simulink model "sysgenMRIDemo"  (Simulink 7.7)
settings: Solver=VariableStepDiscrete  StartTime=0.0  StopTime=inf  RelTol=1e-3
PreLoadFcn:
  | sysgenMRIDemo_PreloadFcn
InitFcn:
  | xlFrameDisplay;
undefined symbols (not defined in the file or in its folder): a, b, c_image_cols, c_image_rows, c_num_fstores, c_swathe_size, sysgenMRIDemo_data_imag_channel, xlFrameDisplay
libraries: xbsIndex_r4 x297, dspsrcs4 x3, xbsCopyrightNotice_r4 x1, simulink x1
(part 3 of 3)

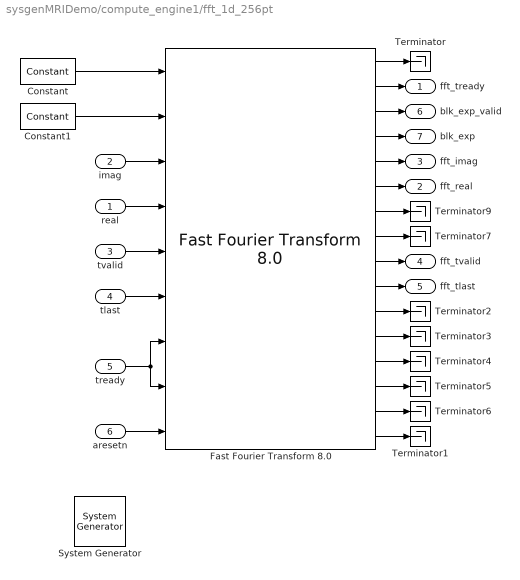
== system sysgenMRIDemo/compute_engine1/fft_1d_256pt ==
  real : Inport
  imag : Inport  Port=2
  tvalid : Inport  Port=3
  tlast : Inport  Port=4
  tready : Inport  Port=5
  aresetn : Inport  Port=6
  " System Generator" : xbsIndex_r4/ System Generator  Tag=genX  SystemSampleTime=-1  xilinxfamily=virtex6  part=xc6vlx240t  speed=-1  package=ff1156  synthesis_tool=XST  clock_wrapper=Clock Enables  directory=./netlist  proj_type=Project Navigator  Synth_file=XST Defaults  Impl_file=ISE Defaults  testbench=off  simulink_period=1  sysclk_period=10  dcm_input_clock_period=10  incr_netlist=off  trim_vbits=Everywhere in SubSystem  dbl_ovrd=According to Block Masks  core_generation=According to Block Masks  run_coregen=off  deprecated_control=off  eval_field=0  block_type=sysgen
      settings: block_version=12.3
  Constant : xbsIndex_r4/Constant  const=1  gui_display_data_type=Fixed-point  arith_type=Unsigned  n_bits=1  bin_pt=0  preci_type=Single  exp_width=8  frac_width=24  explicit_period=on  period=1  equ=P=C  opselect=C  inp2=PCIN>>17  opr=+  inp1=P  carry=CIN  dbl_ovrd=off  block_type=constant
      settings: block_version=12.3
  Constant1 : xbsIndex_r4/Constant  const=0  gui_display_data_type=Fixed-point  arith_type=Boolean  n_bits=16  bin_pt=14  preci_type=Single  exp_width=8  frac_width=24  explicit_period=on  period=1  equ=P=C  opselect=C  inp2=PCIN>>17  opr=+  inp1=P  carry=CIN  dbl_ovrd=off  block_type=constant
      settings: block_version=12.3
  "Fast Fourier Transform 8.0 " : xbsIndex_r4/Fast Fourier Transform 8.0   transform_length=256  target_clock_frequency=250  target_data_throughput=250  implementation_options=automatically_select  run_time_configurable_transform_length=off  phase_factor_width=16  scaling_options=block_floating_point  rounding_modes=truncation  aclken=off  aresetn=on  cyclic_prefix_insertion=off  output_ordering=natural_order  throttle_scheme=nonrealtime  xk_index=on  ovflo=off  trim_axipin_name=on  memory_options_data=block_ram  memory_options_phase_factors=block_ram  number_of_stages_using_block_ram_for_data_and_phase_factors=3  memory_options_reorder=block_ram  memory_options_hybrid=off  complex_mult_type=use_mults_resources  butterfly_type=use_luts  channels=1  input_ordering=natural_order  input_width=16  simulation_model=fftv8_CModel:fftv8_cmodel  ip_name=Fast Fourier Transform  ip_version=8.0  dsptool_ready=true  ipcore_usecache=true  ipcore_useipmodelcache=true  wrapper_available=true  port_translation_map={ 'aclken' => 'en', 'aresetn' => 'rst'}  block_type=xfft_v8_0
      settings: block_version=12.3
  Terminator{,1..7,9} (9 alike) : Terminator
  fft_tready : Outport
  fft_real : Outport  Port=2
  fft_imag : Outport  Port=3
  fft_tvalid : Outport  Port=4
  fft_tlast : Outport  Port=5
  blk_exp_valid : Outport  Port=6
  blk_exp : Outport  Port=7
  wires:
  "Fast Fourier Transform 8.0 "/16 -> Terminator1/1
  "Fast Fourier Transform 8.0 "/15 -> Terminator6/1
  "Fast Fourier Transform 8.0 "/14 -> Terminator5/1
  "Fast Fourier Transform 8.0 "/13 -> Terminator4/1
  "Fast Fourier Transform 8.0 "/12 -> Terminator3/1
  "Fast Fourier Transform 8.0 "/11 -> Terminator2/1
  "Fast Fourier Transform 8.0 "/10 -> fft_tlast/1
  "Fast Fourier Transform 8.0 "/9 -> fft_tvalid/1
  "Fast Fourier Transform 8.0 "/8 -> Terminator7/1
  "Fast Fourier Transform 8.0 "/7 -> Terminator9/1
  "Fast Fourier Transform 8.0 "/6 -> fft_real/1
  "Fast Fourier Transform 8.0 "/5 -> fft_imag/1
  "Fast Fourier Transform 8.0 "/4 -> blk_exp/1
  "Fast Fourier Transform 8.0 "/3 -> blk_exp_valid/1
  "Fast Fourier Transform 8.0 "/2 -> fft_tready/1
  "Fast Fourier Transform 8.0 "/1 -> Terminator/1
  aresetn/1 -> "Fast Fourier Transform 8.0 "/9
  tready/1 -> "Fast Fourier Transform 8.0 "/8, "Fast Fourier Transform 8.0 "/7
  tlast/1 -> "Fast Fourier Transform 8.0 "/6
  tvalid/1 -> "Fast Fourier Transform 8.0 "/5
  real/1 -> "Fast Fourier Transform 8.0 "/4
  imag/1 -> "Fast Fourier Transform 8.0 "/3
  Constant1/1 -> "Fast Fourier Transform 8.0 "/2
  Constant/1 -> "Fast Fourier Transform 8.0 "/1

== system sysgenMRIDemo/image_Src1/Subsystem ==
  Enable : EnablePort  PropagateVarSize=During execution
  Imag Channel : dspsrcs4/Signal From Workspace  SystemSampleTime=-1  X=sysgenMRIDemo_data_imag_channel  Ts=1  nsamps=1  OutputAfterFinalValue=Setting to zero  ignoreOrWarnInputAndFrameLengths=off
  Imag Channel1 : dspsrcs4/Signal From Workspace  SystemSampleTime=-1  X=ones(1,length(sysgenMRIDemo_data_imag_channel))  Ts=1  nsamps=1  OutputAfterFinalValue=Setting to zero  ignoreOrWarnInputAndFrameLengths=off
  Real Channel : dspsrcs4/Signal From Workspace  SystemSampleTime=-1  X=sysgenMRIDemo_data_real_channel  Ts=1  nsamps=1  OutputAfterFinalValue=Setting to zero  ignoreOrWarnInputAndFrameLengths=off
  MriReal : Outport
  MriImag : Outport  Port=2
  MriDataValid : Outport  Port=3
  wires:
  Imag Channel/1 -> MriImag/1
  Real Channel/1 -> MriReal/1
  Imag Channel1/1 -> MriDataValid/1

== system sysgenMRIDemo/Provide Register Data1/MM2S and S2MM Control Register Update/VDMA_Control_Register_Addresses ==
  rst : Inport
  en : Inport  Port=2
  ROM : xbsIndex_r4/ROM  depth=length(c_sequence)  initVector=c_sequence  distributed_mem=Distributed memory  rst=off  init_reg=0  en=off  latency=0  gui_display_data_type=Fixed-point  arith_type=Unsigned  n_bits=32  bin_pt=0  preci_type=Single  exp_width=8  frac_width=24  dbl_ovrd=off  optimize=Area  use_rpm=on  block_type=sprom
      settings: block_version=12.3
  count_down1 : Subsystem  mask{init_val=length(c_sequence)-1}
      mask prompts: init_val "Initial Value"
  seq : Outport
  wires:
  count_down1/1(cnt) -> ROM/1
  rst/1 -> count_down1/1(rst)
  ROM/1 -> seq/1
  en/1 -> count_down1/2(en)

== system sysgenMRIDemo/Provide Register Data1/MM2S and S2MM Control Register Update/VDMA_Control_Register_Addresses1 ==
  rst : Inport
  en : Inport  Port=2
  ROM : xbsIndex_r4/ROM  depth=length(c_sequence)  initVector=c_sequence  distributed_mem=Distributed memory  rst=off  init_reg=0  en=off  latency=0  gui_display_data_type=Fixed-point  arith_type=Unsigned  n_bits=32  bin_pt=0  preci_type=Single  exp_width=8  frac_width=24  dbl_ovrd=off  optimize=Area  use_rpm=on  block_type=sprom
      settings: block_version=12.3
  count_down1 : Subsystem  mask{init_val=length(c_sequence)-1}
      mask prompts: init_val "Initial Value"
  seq : Outport
  wires:
  count_down1/1(cnt) -> ROM/1
  rst/1 -> count_down1/1(rst)
  ROM/1 -> seq/1
  en/1 -> count_down1/2(en)

== system sysgenMRIDemo/Provide Register Data1/MM2S and S2MM Control Register Update/pulse_gen_we ==
  d : Inport
  rst : Inport  Port=2
  en : Inport  Port=3
  Register{,1..7} (8 alike) : xbsIndex_r4/Register  init=1  rst=on  en=on  dbl_ovrd=off  block_type=register
      settings: block_version=12.3
  q : Outport
  wires:
  Register6/1 -> Register7/1
  Register5/1 -> Register6/1
  Register4/1 -> Register5/1
  Register3/1 -> Register4/1
  Register7/1 -> q/1
  Register2/1 -> Register3/1
  en/1 -> Register7/3, Register6/3, Register5/3, Register4/3, Register3/3, Register2/3, Register1/3, Register/3
  rst/1 -> Register7/2, Register6/2, Register5/2, Register4/2, Register3/2, Register2/2, Register1/2, Register/2
  d/1 -> Register/1
  Register/1 -> Register1/1
  Register1/1 -> Register2/1

== system sysgenMRIDemo/Provide Register Data1/MM2S and S2MM Control Register Update/pulse_gen_we1 ==
  d : Inport
  rst : Inport  Port=2
  en : Inport  Port=3
  Register{,1..7} (8 alike) : xbsIndex_r4/Register  init=0  rst=on  en=on  dbl_ovrd=off  block_type=register
      settings: block_version=12.3
  q : Outport
  wires:
  Register6/1 -> Register7/1
  Register5/1 -> Register6/1
  Register3/1 -> Register4/1
  Register4/1 -> Register5/1
  Register1/1 -> Register2/1
  Register/1 -> Register1/1
  d/1 -> Register/1
  rst/1 -> Register/2, Register1/2, Register7/2, Register6/2, Register5/2, Register4/2, Register3/2, Register2/2
  en/1 -> Register/3, Register1/3, Register2/3, Register3/3, Register4/3, Register5/3, Register6/3, Register7/3
  Register2/1 -> Register3/1
  Register7/1 -> q/1

== system sysgenMRIDemo/Provide Register Data1/MM2S and S2MM Control Register Update/pulse_gen_we2 ==
  d : Inport
  rst : Inport  Port=2
  en : Inport  Port=3
  Register{,1..3} (4 alike) : xbsIndex_r4/Register  init=1  rst=on  en=on  dbl_ovrd=off  block_type=register
      settings: block_version=12.3
  q : Outport
  wires:
  Register3/1 -> q/1
  Register2/1 -> Register3/1
  en/1 -> Register2/3, Register3/3, Register1/3, Register/3
  rst/1 -> Register2/2, Register3/2, Register1/2, Register/2
  d/1 -> Register/1
  Register/1 -> Register1/1
  Register1/1 -> Register2/1

== system sysgenMRIDemo/Provide Register Data1/MM2S and S2MM Control Register Update/pulse_gen_we3 ==
  d : Inport
  rst : Inport  Port=2
  en : Inport  Port=3
  Register{,1..3} (4 alike) : xbsIndex_r4/Register  init=0  rst=on  en=on  dbl_ovrd=off  block_type=register
      settings: block_version=12.3
  q : Outport
  wires:
  Register1/1 -> Register2/1
  Register/1 -> Register1/1
  d/1 -> Register/1
  rst/1 -> Register/2, Register1/2, Register2/2, Register3/2
  en/1 -> Register/3, Register1/3, Register2/3, Register3/3
  Register2/1 -> Register3/1
  Register3/1 -> q/1

== system sysgenMRIDemo/Provide Register Data1/MM2S and S2MM Control Register Update/register_sequence ==
  rst : Inport
  en : Inport  Port=2
  ROM : xbsIndex_r4/ROM  depth=length(c_sequence)  initVector=c_sequence  distributed_mem=Distributed memory  rst=off  init_reg=0  en=off  latency=0  gui_display_data_type=Fixed-point  arith_type=Unsigned  n_bits=32  bin_pt=0  preci_type=Single  exp_width=8  frac_width=24  dbl_ovrd=off  optimize=Area  use_rpm=on  block_type=sprom
      settings: block_version=12.3
  count_down1 : Subsystem  mask{init_val=length(c_sequence)-1}
      mask prompts: init_val "Initial Value"
  seq : Outport
  wires:
  count_down1/1(cnt) -> ROM/1
  rst/1 -> count_down1/1(rst)
  ROM/1 -> seq/1
  en/1 -> count_down1/2(en)

== system sysgenMRIDemo/Provide Register Data1/MM2S and S2MM Control Register Update/register_sequence1 ==
  rst : Inport
  en : Inport  Port=2
  ROM : xbsIndex_r4/ROM  depth=length(c_sequence)  initVector=c_sequence  distributed_mem=Distributed memory  rst=off  init_reg=0  en=off  latency=0  gui_display_data_type=Fixed-point  arith_type=Unsigned  n_bits=32  bin_pt=0  preci_type=Single  exp_width=8  frac_width=24  dbl_ovrd=off  optimize=Area  use_rpm=on  block_type=sprom
      settings: block_version=12.3
  count_down1 : Subsystem  mask{init_val=length(c_sequence)-1}
      mask prompts: init_val "Initial Value"
  seq : Outport
  wires:
  count_down1/1(cnt) -> ROM/1
  rst/1 -> count_down1/1(rst)
  ROM/1 -> seq/1
  en/1 -> count_down1/2(en)

== system sysgenMRIDemo/Provide Register Data1/S2MM Control Register Update/VDMA_Control_Register_Addresses ==
  rst : Inport
  en : Inport  Port=2
  ROM : xbsIndex_r4/ROM  depth=length(c_sequence)  initVector=c_sequence  distributed_mem=Distributed memory  rst=off  init_reg=0  en=off  latency=0  gui_display_data_type=Fixed-point  arith_type=Unsigned  n_bits=32  bin_pt=0  preci_type=Single  exp_width=8  frac_width=24  dbl_ovrd=off  optimize=Area  use_rpm=on  block_type=sprom
      settings: block_version=12.3
  count_down1 : Subsystem  mask{init_val=length(c_sequence)-1}
      mask prompts: init_val "Initial Value"
  seq : Outport
  wires:
  count_down1/1(cnt) -> ROM/1
  rst/1 -> count_down1/1(rst)
  ROM/1 -> seq/1
  en/1 -> count_down1/2(en)

== system sysgenMRIDemo/Provide Register Data1/S2MM Control Register Update/VDMA_Control_Register_Data2 ==
  rst : Inport
  en : Inport  Port=2
  ROM : xbsIndex_r4/ROM  depth=length(c_sequence)  initVector=c_sequence  distributed_mem=Distributed memory  rst=off  init_reg=0  en=off  latency=0  gui_display_data_type=Fixed-point  arith_type=Unsigned  n_bits=32  bin_pt=0  preci_type=Single  exp_width=8  frac_width=24  dbl_ovrd=off  optimize=Area  use_rpm=on  block_type=sprom
      settings: block_version=12.3
  count_down1 : Subsystem  mask{init_val=length(c_sequence)-1}
      mask prompts: init_val "Initial Value"
  seq : Outport
  wires:
  count_down1/1(cnt) -> ROM/1
  rst/1 -> count_down1/1(rst)
  ROM/1 -> seq/1
  en/1 -> count_down1/2(en)

== system sysgenMRIDemo/Provide Register Data1/S2MM Control Register Update/pulse_gen_re ==
  d : Inport
  rst : Inport  Port=2
  en : Inport  Port=3
  Register{,1..3} (4 alike) : xbsIndex_r4/Register  init=0  rst=on  en=on  dbl_ovrd=off  block_type=register
      settings: block_version=12.3
  q : Outport
  wires:
  Register3/1 -> q/1
  Register2/1 -> Register3/1
  Register1/1 -> Register2/1
  Register/1 -> Register1/1
  d/1 -> Register/1
  rst/1 -> Register/2, Register3/2, Register2/2, Register1/2
  en/1 -> Register/3, Register3/3, Register2/3, Register1/3

== system sysgenMRIDemo/Provide Register Data1/S2MM Control Register Update/pulse_gen_we ==
  d : Inport
  rst : Inport  Port=2
  en : Inport  Port=3
  Register{,1..3} (4 alike) : xbsIndex_r4/Register  init=1  rst=on  en=on  dbl_ovrd=off  block_type=register
      settings: block_version=12.3
  q : Outport
  wires:
  Register3/1 -> q/1
  Register2/1 -> Register3/1
  en/1 -> Register3/3, Register2/3, Register1/3, Register/3
  rst/1 -> Register3/2, Register2/2, Register1/2, Register/2
  d/1 -> Register/1
  Register/1 -> Register1/1
  Register1/1 -> Register2/1

== system sysgenMRIDemo/Provide Register Data1/MM2S and S2MM Control Register Update/VDMA_Control_Register_Addresses/count_down1 ==
  rst : Inport
  en : Inport  Port=2
  Constant3 : xbsIndex_r4/Constant  const=0  gui_display_data_type=Fixed-point  arith_type=Unsigned  n_bits=ceil(ceil( (c_image_rows/c_swathe_size) / c_num_fstores) + 1)  bin_pt=0  preci_type=Single  exp_width=8  frac_width=24  explicit_period=off  period=1  equ=P=C  opselect=C  inp2=PCIN>>17  opr=+  inp1=P  carry=CIN  dbl_ovrd=off  block_type=constant
      settings: block_version=12.3
  Counter : xbsIndex_r4/Counter  cnt_type=Count Limited  cnt_to=0  operation=Down  start_count=init_val  cnt_by_val=1  arith_type=Unsigned  n_bits=ceil(log2(init_val + 1))  bin_pt=0  load_pin=off  rst=on  en=on  explicit_period=on  period=1  dbl_ovrd=off  use_behavioral_HDL=off  implementation=Fabric  block_type=counter
      settings: block_version=12.3
  Expression : xbsIndex_r4/Expression  expression=a & b  align_bp=on  en=off  latency=0  precision=Full  arith_type=Unsigned  n_bits=16  bin_pt=0  dbl_ovrd=off  block_type=expr
      settings: block_version=12.3
  Relational1 : xbsIndex_r4/Relational  mode=a!=b  en=off  latency=0  dbl_ovrd=off  block_type=relational
      settings: block_version=12.3
  cnt : Outport
  wires:
  en/1 -> Expression/2
  Relational1/1 -> Expression/1
  Constant3/1 -> Relational1/2
  Counter/1 -> cnt/1, Relational1/1
  Expression/1 -> Counter/2
  rst/1 -> Counter/1

== system sysgenMRIDemo/Provide Register Data1/MM2S and S2MM Control Register Update/VDMA_Control_Register_Addresses1/count_down1 ==
  rst : Inport
  en : Inport  Port=2
  Constant3 : xbsIndex_r4/Constant  const=0  gui_display_data_type=Fixed-point  arith_type=Unsigned  n_bits=ceil(ceil( (c_image_rows/c_swathe_size) / c_num_fstores) + 1)  bin_pt=0  preci_type=Single  exp_width=8  frac_width=24  explicit_period=off  period=1  equ=P=C  opselect=C  inp2=PCIN>>17  opr=+  inp1=P  carry=CIN  dbl_ovrd=off  block_type=constant
      settings: block_version=12.3
  Counter : xbsIndex_r4/Counter  cnt_type=Count Limited  cnt_to=0  operation=Down  start_count=init_val  cnt_by_val=1  arith_type=Unsigned  n_bits=ceil(log2(init_val + 1))  bin_pt=0  load_pin=off  rst=on  en=on  explicit_period=on  period=1  dbl_ovrd=off  use_behavioral_HDL=off  implementation=Fabric  block_type=counter
      settings: block_version=12.3
  Expression : xbsIndex_r4/Expression  expression=a & b  align_bp=on  en=off  latency=0  precision=Full  arith_type=Unsigned  n_bits=16  bin_pt=0  dbl_ovrd=off  block_type=expr
      settings: block_version=12.3
  Relational1 : xbsIndex_r4/Relational  mode=a!=b  en=off  latency=0  dbl_ovrd=off  block_type=relational
      settings: block_version=12.3
  cnt : Outport
  wires:
  en/1 -> Expression/2
  Relational1/1 -> Expression/1
  Constant3/1 -> Relational1/2
  Counter/1 -> cnt/1, Relational1/1
  Expression/1 -> Counter/2
  rst/1 -> Counter/1

== system sysgenMRIDemo/Provide Register Data1/MM2S and S2MM Control Register Update/register_sequence/count_down1 ==
  rst : Inport
  en : Inport  Port=2
  Constant3 : xbsIndex_r4/Constant  const=0  gui_display_data_type=Fixed-point  arith_type=Unsigned  n_bits=ceil(ceil( (c_image_rows/c_swathe_size) / c_num_fstores) + 1)  bin_pt=0  preci_type=Single  exp_width=8  frac_width=24  explicit_period=off  period=1  equ=P=C  opselect=C  inp2=PCIN>>17  opr=+  inp1=P  carry=CIN  dbl_ovrd=off  block_type=constant
      settings: block_version=12.3
  Counter : xbsIndex_r4/Counter  cnt_type=Count Limited  cnt_to=0  operation=Down  start_count=init_val  cnt_by_val=1  arith_type=Unsigned  n_bits=ceil(log2(init_val + 1))  bin_pt=0  load_pin=off  rst=on  en=on  explicit_period=on  period=1  dbl_ovrd=off  use_behavioral_HDL=off  implementation=Fabric  block_type=counter
      settings: block_version=12.3
  Expression : xbsIndex_r4/Expression  expression=a & b  align_bp=on  en=off  latency=0  precision=Full  arith_type=Unsigned  n_bits=16  bin_pt=0  dbl_ovrd=off  block_type=expr
      settings: block_version=12.3
  Relational1 : xbsIndex_r4/Relational  mode=a!=b  en=off  latency=0  dbl_ovrd=off  block_type=relational
      settings: block_version=12.3
  cnt : Outport
  wires:
  en/1 -> Expression/2
  Relational1/1 -> Expression/1
  Constant3/1 -> Relational1/2
  Counter/1 -> cnt/1, Relational1/1
  Expression/1 -> Counter/2
  rst/1 -> Counter/1

== system sysgenMRIDemo/Provide Register Data1/MM2S and S2MM Control Register Update/register_sequence1/count_down1 ==
  rst : Inport
  en : Inport  Port=2
  Constant3 : xbsIndex_r4/Constant  const=0  gui_display_data_type=Fixed-point  arith_type=Unsigned  n_bits=ceil(ceil( (c_image_rows/c_swathe_size) / c_num_fstores) + 1)  bin_pt=0  preci_type=Single  exp_width=8  frac_width=24  explicit_period=off  period=1  equ=P=C  opselect=C  inp2=PCIN>>17  opr=+  inp1=P  carry=CIN  dbl_ovrd=off  block_type=constant
      settings: block_version=12.3
  Counter : xbsIndex_r4/Counter  cnt_type=Count Limited  cnt_to=0  operation=Down  start_count=init_val  cnt_by_val=1  arith_type=Unsigned  n_bits=ceil(log2(init_val + 1))  bin_pt=0  load_pin=off  rst=on  en=on  explicit_period=on  period=1  dbl_ovrd=off  use_behavioral_HDL=off  implementation=Fabric  block_type=counter
      settings: block_version=12.3
  Expression : xbsIndex_r4/Expression  expression=a & b  align_bp=on  en=off  latency=0  precision=Full  arith_type=Unsigned  n_bits=16  bin_pt=0  dbl_ovrd=off  block_type=expr
      settings: block_version=12.3
  Relational1 : xbsIndex_r4/Relational  mode=a!=b  en=off  latency=0  dbl_ovrd=off  block_type=relational
      settings: block_version=12.3
  cnt : Outport
  wires:
  en/1 -> Expression/2
  Relational1/1 -> Expression/1
  Constant3/1 -> Relational1/2
  Counter/1 -> cnt/1, Relational1/1
  Expression/1 -> Counter/2
  rst/1 -> Counter/1

== system sysgenMRIDemo/Provide Register Data1/S2MM Control Register Update/VDMA_Control_Register_Addresses/count_down1 ==
  rst : Inport
  en : Inport  Port=2
  Constant3 : xbsIndex_r4/Constant  const=0  gui_display_data_type=Fixed-point  arith_type=Unsigned  n_bits=ceil(ceil( (c_image_rows/c_swathe_size) / c_num_fstores) + 1)  bin_pt=0  preci_type=Single  exp_width=8  frac_width=24  explicit_period=off  period=1  equ=P=C  opselect=C  inp2=PCIN>>17  opr=+  inp1=P  carry=CIN  dbl_ovrd=off  block_type=constant
      settings: block_version=12.3
  Counter : xbsIndex_r4/Counter  cnt_type=Count Limited  cnt_to=0  operation=Down  start_count=init_val  cnt_by_val=1  arith_type=Unsigned  n_bits=ceil(log2(init_val + 1))  bin_pt=0  load_pin=off  rst=on  en=on  explicit_period=on  period=1  dbl_ovrd=off  use_behavioral_HDL=off  implementation=Fabric  block_type=counter
      settings: block_version=12.3
  Expression : xbsIndex_r4/Expression  expression=a & b  align_bp=on  en=off  latency=0  precision=Full  arith_type=Unsigned  n_bits=16  bin_pt=0  dbl_ovrd=off  block_type=expr
      settings: block_version=12.3
  Relational1 : xbsIndex_r4/Relational  mode=a!=b  en=off  latency=0  dbl_ovrd=off  block_type=relational
      settings: block_version=12.3
  cnt : Outport
  wires:
  en/1 -> Expression/2
  Relational1/1 -> Expression/1
  Constant3/1 -> Relational1/2
  Counter/1 -> cnt/1, Relational1/1
  Expression/1 -> Counter/2
  rst/1 -> Counter/1

== system sysgenMRIDemo/Provide Register Data1/S2MM Control Register Update/VDMA_Control_Register_Data2/count_down1 ==
  rst : Inport
  en : Inport  Port=2
  Constant3 : xbsIndex_r4/Constant  const=0  gui_display_data_type=Fixed-point  arith_type=Unsigned  n_bits=ceil(ceil( (c_image_rows/c_swathe_size) / c_num_fstores) + 1)  bin_pt=0  preci_type=Single  exp_width=8  frac_width=24  explicit_period=off  period=1  equ=P=C  opselect=C  inp2=PCIN>>17  opr=+  inp1=P  carry=CIN  dbl_ovrd=off  block_type=constant
      settings: block_version=12.3
  Counter : xbsIndex_r4/Counter  cnt_type=Count Limited  cnt_to=0  operation=Down  start_count=init_val  cnt_by_val=1  arith_type=Unsigned  n_bits=ceil(log2(init_val + 1))  bin_pt=0  load_pin=off  rst=on  en=on  explicit_period=on  period=1  dbl_ovrd=off  use_behavioral_HDL=off  implementation=Fabric  block_type=counter
      settings: block_version=12.3
  Expression : xbsIndex_r4/Expression  expression=a & b  align_bp=on  en=off  latency=0  precision=Full  arith_type=Unsigned  n_bits=16  bin_pt=0  dbl_ovrd=off  block_type=expr
      settings: block_version=12.3
  Relational1 : xbsIndex_r4/Relational  mode=a!=b  en=off  latency=0  dbl_ovrd=off  block_type=relational
      settings: block_version=12.3
  cnt : Outport
  wires:
  en/1 -> Expression/2
  Relational1/1 -> Expression/1
  Constant3/1 -> Relational1/2
  Counter/1 -> cnt/1, Relational1/1
  Expression/1 -> Counter/2
  rst/1 -> Counter/1
